simulink model "DLC"  (Simulink 7.5)
settings: Solver=ode3  StartTime=0.0  StopTime=5  FixedStep=5e-005  RelTol=1e-3
libraries: simulink x2, powerlib_extras x1, powerlib x1
settings Model: Creator=lm  LastModifiedBy=lm

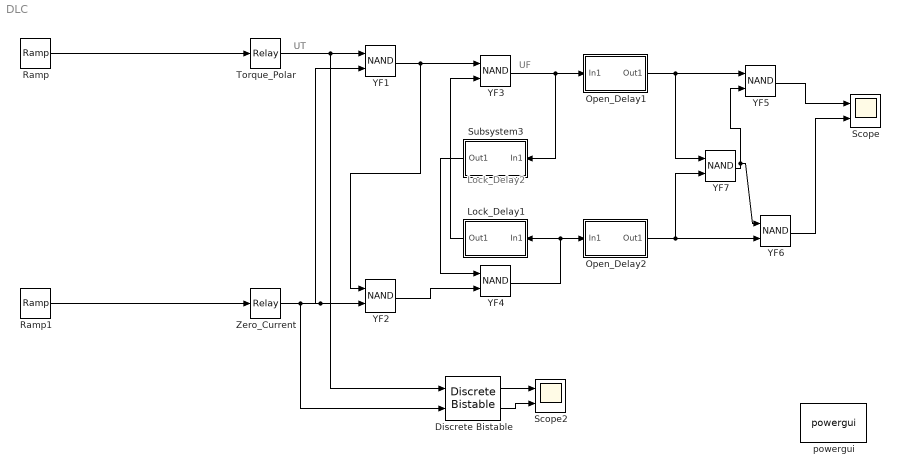
== system DLC ==
  note: Lock_Delay2
  note: UF
  note: UT
  Discrete Bistable : powerlib_extras/Discrete  Control Blocks/Discrete Bistable  DialogController=POWERSYS.PowerSysDialog  SystemSampleTime=-1  SPSpriority=Set  ic=0  Ts=50e-6
  Lock_Delay1 : Subsystem
  Open_Delay1 : Subsystem
  Open_Delay2 : Subsystem
  Ramp : simulink/Sources/Ramp  SystemSampleTime=-1  slope=0  start=0  X0=10
  Ramp1 : simulink/Sources/Ramp  SystemSampleTime=-1  slope=0  start=0  X0=2
  Scope : Scope  NumInputPorts=2
      settings: YMin=-5~-5  YMax=5~5
  Scope2 : Scope  NumInputPorts=2
      settings: TimeRange=20  YMin=-5~2  YMax=5~4  SaveName=ScopeData2
  Subsystem3 : Subsystem
  Torque_Polar : Relay  OnSwitchValue=0.001  OffSwitchValue=-0.001  OutDataType=fixdt(1, 16)  OutScaling=2^0
  YF1 : Logic  Operator=NAND  AllPortsSameDT=off  LogicDataType=fixdt(0, 8)
  YF{2..7} (6 alike) : Logic  Operator=NAND  AllPortsSameDT=off  OutDataTypeMode=boolean  LogicDataType=fixdt(0, 8)  OutDataTypeStr=boolean
  Zero_Current : Relay  OnSwitchValue=0.5  OffSwitchValue=0.01  OnOutputValue=0  OffOutputValue=1  OutDataType=fixdt(1, 16)  OutScaling=2^0
  powergui : powerlib/powergui  Priority=1  SystemSampleTime=-1  SimulationMode=Discrete  SampleTime=50e-6  frequency=60  SPID=off  DisableSnubberDevices=off  DisableRonSwitches=off  DisableVfSwitches=off  SwTol=0  Interpol=off  frequencyindice=60  echomessages=off  HookPort=off  DisplayEquations=off  FunctionMessages=off  EnableUseOfTLC=off  x0status=blocks  RestoreLinks=warning  ResistiveCurrentMeasurement=off  Ylog=off  Xlog=on  ShowGrid=off  save=off  variable=ZData  ZoomFFT=off  StartTime=0.0  cycles=1  DisplayStyle=1  FreqAxis=off  MaxFrequency=1000  frequencyindicesteady=1  display=off  methode=off
  wires:
  Torque_Polar/1 -> YF1/1, Discrete Bistable/1
  Zero_Current/1 -> YF1/2, YF2/2, Discrete Bistable/2
  YF1/1 -> YF2/1, YF3/1
  Lock_Delay1/1(Out1) -> YF3/2
  Subsystem3/1(Out1) -> YF4/1
  YF2/1 -> YF4/2
  YF4/1 -> Lock_Delay1/1(In1), Open_Delay2/1(In1)
  YF3/1 -> Subsystem3/1(In1), Open_Delay1/1(In1)
  Open_Delay1/1(Out1) -> YF7/1, YF5/1
  Open_Delay2/1(Out1) -> YF7/2, YF6/2
  YF7/1 -> YF5/2, YF6/1
  YF5/1 -> Scope/1
  YF6/1 -> Scope/2
  Ramp/1 -> Torque_Polar/1
  Ramp1/1 -> Zero_Current/1
  Discrete Bistable/1 -> Scope2/1
  Discrete Bistable/2 -> Scope2/2

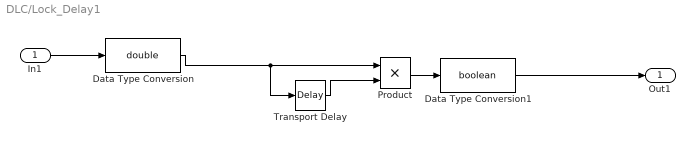
== system DLC/Lock_Delay1 ==
  In1 : Inport  OutDataType=fixdt(1, 16)  OutScaling=2^0
  Data Type Conversion : DataTypeConversion  OutDataTypeMode=double  OutDataType=fixdt(1, 16)  OutScaling=2^0  OutDataTypeStr=double
  Data Type Conversion1 : DataTypeConversion  OutDataTypeMode=boolean  OutDataType=fixdt(1, 16)  OutScaling=2^0  OutDataTypeStr=boolean
  Product : Product  OutDataType=fixdt(1, 16)  OutScaling=2^0  RndMeth=Zero
  Transport Delay : TransportDelay  DelayTime=3e-3
  Out1 : Outport  OutDataType=fixdt(1, 16)  OutScaling=2^0
  wires:
  Data Type Conversion1/1 -> Out1/1
  Product/1 -> Data Type Conversion1/1
  In1/1 -> Data Type Conversion/1
  Data Type Conversion/1 -> Product/1, Transport Delay/1
  Transport Delay/1 -> Product/2

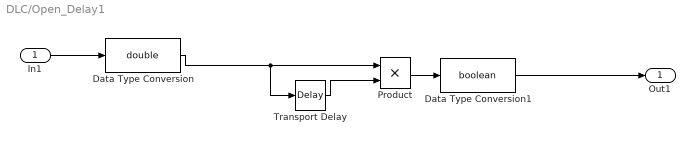
== system DLC/Open_Delay1 ==
  In1 : Inport  OutDataType=fixdt(1, 16)  OutScaling=2^0
  Data Type Conversion : DataTypeConversion  OutDataTypeMode=double  OutDataType=fixdt(1, 16)  OutScaling=2^0  OutDataTypeStr=double
  Data Type Conversion1 : DataTypeConversion  OutDataTypeMode=boolean  OutDataType=fixdt(1, 16)  OutScaling=2^0  OutDataTypeStr=boolean
  Product : Product  OutDataType=fixdt(1, 16)  OutScaling=2^0  RndMeth=Zero
  Transport Delay : TransportDelay  DelayTime=7e-3
  Out1 : Outport  OutDataType=fixdt(1, 16)  OutScaling=2^0
  wires:
  Data Type Conversion1/1 -> Out1/1
  Product/1 -> Data Type Conversion1/1
  In1/1 -> Data Type Conversion/1
  Data Type Conversion/1 -> Product/1, Transport Delay/1
  Transport Delay/1 -> Product/2

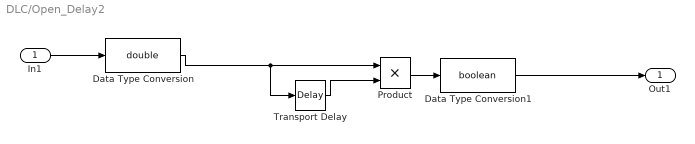
== system DLC/Open_Delay2 ==
  In1 : Inport  OutDataType=fixdt(1, 16)  OutScaling=2^0
  Data Type Conversion : DataTypeConversion  OutDataTypeMode=double  OutDataType=fixdt(1, 16)  OutScaling=2^0  OutDataTypeStr=double
  Data Type Conversion1 : DataTypeConversion  OutDataTypeMode=boolean  OutDataType=fixdt(1, 16)  OutScaling=2^0  OutDataTypeStr=boolean
  Product : Product  OutDataType=fixdt(1, 16)  OutScaling=2^0  RndMeth=Zero
  Transport Delay : TransportDelay  DelayTime=7e-3
  Out1 : Outport  OutDataType=fixdt(1, 16)  OutScaling=2^0
  wires:
  Transport Delay/1 -> Product/2
  Data Type Conversion/1 -> Transport Delay/1, Product/1
  In1/1 -> Data Type Conversion/1
  Product/1 -> Data Type Conversion1/1
  Data Type Conversion1/1 -> Out1/1

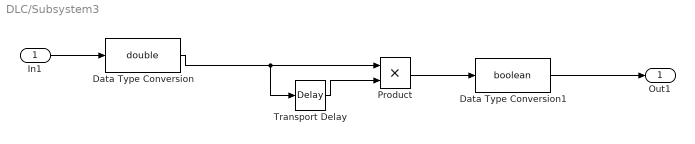
== system DLC/Subsystem3 ==
  In1 : Inport  OutDataType=fixdt(1, 16)  OutScaling=2^0
  Data Type Conversion : DataTypeConversion  OutDataTypeMode=double  OutDataType=fixdt(1, 16)  OutScaling=2^0  OutDataTypeStr=double
  Data Type Conversion1 : DataTypeConversion  OutDataTypeMode=boolean  OutDataType=fixdt(1, 16)  OutScaling=2^0  OutDataTypeStr=boolean
  Product : Product  OutDataType=fixdt(1, 16)  OutScaling=2^0  RndMeth=Zero
  Transport Delay : TransportDelay  DelayTime=3e-3
  Out1 : Outport  OutDataType=fixdt(1, 16)  OutScaling=2^0
  wires:
  Transport Delay/1 -> Product/2
  Data Type Conversion/1 -> Transport Delay/1, Product/1
  In1/1 -> Data Type Conversion/1
  Product/1 -> Data Type Conversion1/1
  Data Type Conversion1/1 -> Out1/1
